simulink model "advisordemo2"  (Simulink 5.0)
settings: Solver=FixedStepDiscrete  SolverMode=SingleTasking  StartTime=0.0  StopTime=4  FixedStep=1  RelTol=1e-3  AbsTol=1e-6
libraries: fixpt_lib_4 x4
settings Model: ExecutionOrder=on  CovMetricSettings=d  Creator=andyb  LastModifiedBy=batserve  ExtModeMexFile=no_ext_comm  ExtModeTrigMode=oneshot  ExtModeArmWhenConnect=off  ExtModeAutoUpdateStatusClock=off  RTWExpressionDepthLimit=1  SaveTime=off  SaveOutput=off  LimitDataPoints=off  IntegerOverflowMsg=none  ParameterDowncastMsg=warning  ParameterOverflowMsg=warning  ParameterPrecisionLossMsg=none  RTWInlineParameters=on  ProdHWWordLengths=8,16,16,32  RTWSystemTargetFile=ert.tlc  RTWTemplateMakefile=ert_default_tmf  RTWGenerateCodeOnly=on  RTWOptions="-aCombineOutputUpdateFcns=1 -aEnforceIntegerDowncast=0 -aExtMode=0 -aExtModeTesting=0 -aFoldNonRolledExpr=1 -aForceParamTrailComments=0 -aGenFloatMathFcnCalls=\"ANSI_C\" -aGenerateASAP2=0 -aGenerateComments=1 -aGenerateErtSFunction=0 -aGenerateReport=1 -aGenerateSampleERTMain=0 -aIgnoreCustomStorageClasses=0 -aIncDataTypeInIds=1 -aIncHierarchyInIds=1 -aIncludeMdlTerminateFcn=0 -aInitFltsAndDblsToZero=0 -aInlineInvariantSignals=1 -aInlinedPrmAccess=\"Literals\" -aInsertBlockDesc=0 -aLocalBlockOutputs=1 -aMatFileLogging=0 -aMaxRTWIdLen=31 -aMultiInstanceERTCode=0 -aPrefixModelToSubsysFcnNames=1 -aPurelyIntegerCode=0 -aRTWVerbose=1 -aRollThreshold=5 -aShowEliminatedStatements=0 -aSuppressErrorStatus=1 -aZeroExternalMemoryAtStartup=0 -aZeroInternalMemoryAtStartup=0"

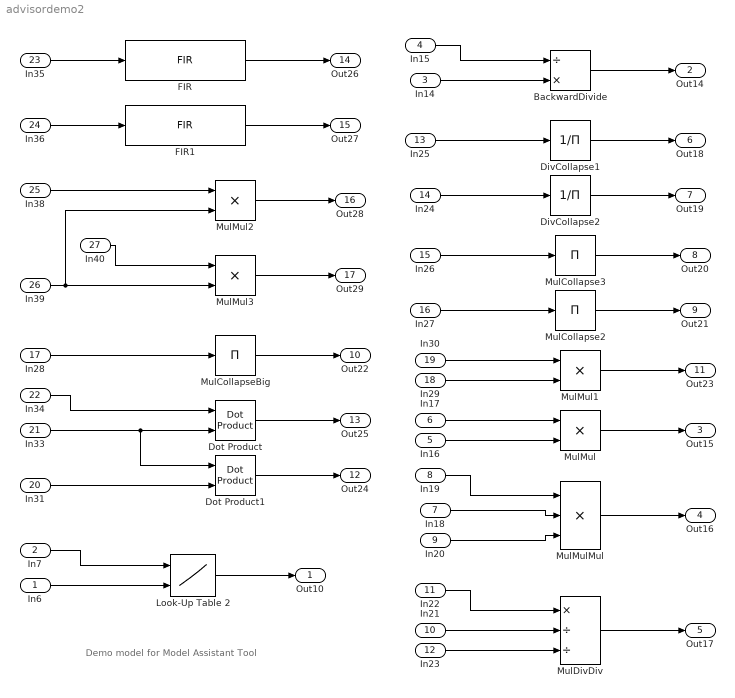
== system advisordemo2 ==
  note: Demo model for Model Assistant Tool
  In6 : Inport  PortDimensions=1  SampleTime=1  ShowAdditionalParam=on  DataType=Specify via dialog  OutScaling=2^-10  Interpolate=off
  In7 : Inport  Port=2  PortDimensions=1  SampleTime=1  ShowAdditionalParam=on  DataType=Specify via dialog  OutScaling=2^-10  Interpolate=off
  In14 : Inport  Port=3  PortDimensions=1  SampleTime=1  ShowAdditionalParam=on  DataType=Specify via dialog  OutScaling=2^-10  Interpolate=off
  In15 : Inport  Port=4  PortDimensions=1  SampleTime=1  ShowAdditionalParam=on  DataType=Specify via dialog  OutScaling=2^-10  Interpolate=off
  In16 : Inport  Port=5  PortDimensions=1  SampleTime=1  ShowAdditionalParam=on  DataType=Specify via dialog  OutDataType=sfix(32)  OutScaling=2^-10  Interpolate=off
  In17 : Inport  Port=6  PortDimensions=1  SampleTime=1  ShowAdditionalParam=on  DataType=Specify via dialog  OutScaling=2^-10  Interpolate=off
  In18 : Inport  Port=7  PortDimensions=1  SampleTime=1  ShowAdditionalParam=on  DataType=Specify via dialog  OutScaling=2^-10  Interpolate=off
  In19 : Inport  Port=8  PortDimensions=1  SampleTime=1  ShowAdditionalParam=on  DataType=Specify via dialog  OutScaling=2^-10  Interpolate=off
  In20 : Inport  Port=9  PortDimensions=1  SampleTime=1  ShowAdditionalParam=on  DataType=Specify via dialog  OutScaling=2^-10  Interpolate=off
  In21 : Inport  Port=10  PortDimensions=1  SampleTime=1  ShowAdditionalParam=on  DataType=Specify via dialog  OutScaling=2^-10  Interpolate=off
  In22 : Inport  Port=11  PortDimensions=1  SampleTime=1  ShowAdditionalParam=on  DataType=Specify via dialog  OutScaling=2^-10  Interpolate=off
  In23 : Inport  Port=12  PortDimensions=1  SampleTime=1  ShowAdditionalParam=on  DataType=Specify via dialog  OutScaling=2^-10  Interpolate=off
  In25 : Inport  Port=13  PortDimensions=1  SampleTime=1  ShowAdditionalParam=on  DataType=Specify via dialog  OutScaling=2^-10  Interpolate=off
  In24 : Inport  Port=14  PortDimensions=2  SampleTime=1  ShowAdditionalParam=on  DataType=Specify via dialog  OutScaling=2^-10  Interpolate=off
  In26 : Inport  Port=15  PortDimensions=3  SampleTime=1  ShowAdditionalParam=on  DataType=Specify via dialog  OutScaling=2^-10  Interpolate=off
  In27 : Inport  Port=16  PortDimensions=2  SampleTime=1  ShowAdditionalParam=on  DataType=Specify via dialog  OutScaling=2^-10  Interpolate=off
  In28 : Inport  Port=17  PortDimensions=2  SampleTime=1  ShowAdditionalParam=on  DataType=Specify via dialog  OutDataType=sfix(32)  OutScaling=2^-10  Interpolate=off
  In29 : Inport  Port=18  PortDimensions=1  SampleTime=1  ShowAdditionalParam=on  DataType=Specify via dialog  OutScaling=2^-10  Interpolate=off
  In30 : Inport  Port=19  PortDimensions=1  SampleTime=1  ShowAdditionalParam=on  DataType=Specify via dialog  OutScaling=2^-10  Interpolate=off
  In31 : Inport  Port=20  PortDimensions=1  SampleTime=1  ShowAdditionalParam=on  DataType=Specify via dialog  OutDataType=sfix(32)  OutScaling=2^-10  Interpolate=off
  In33 : Inport  Port=21  PortDimensions=1  SampleTime=1  ShowAdditionalParam=on  DataType=Specify via dialog  OutScaling=2^-10  Interpolate=off
  In34 : Inport  Port=22  PortDimensions=1  SampleTime=1  ShowAdditionalParam=on  DataType=Specify via dialog  OutScaling=2^-10  Interpolate=off
  In35 : Inport  Port=23  PortDimensions=1  SampleTime=1  ShowAdditionalParam=on  DataType=Specify via dialog  OutDataType=sfix(32)  OutScaling=2^-10  Interpolate=off
  In36 : Inport  Port=24  PortDimensions=1  SampleTime=1  ShowAdditionalParam=on  DataType=Specify via dialog  OutDataType=sfix(32)  OutScaling=2^-10  Interpolate=off
  In38 : Inport  Port=25  PortDimensions=1  SampleTime=1  ShowAdditionalParam=on  DataType=Specify via dialog  OutScaling=1.01 * 2^-10  Interpolate=off
  In39 : Inport  Port=26  PortDimensions=1  SampleTime=1  ShowAdditionalParam=on  DataType=Specify via dialog  OutScaling=2^-10  Interpolate=off
  In40 : Inport  Port=27  PortDimensions=1  SampleTime=1  ShowAdditionalParam=on  DataType=Specify via dialog  OutScaling=[2^-10 1]  Interpolate=off
  BackwardDivide : Product  Inputs=/*  ShowAdditionalParam=on  OutDataTypeMode=Specify via dialog  OutScaling=2^-10
  DivCollapse1 : Product  Inputs=/  ShowAdditionalParam=on  OutDataTypeMode=Specify via dialog  OutScaling=2^-10
  DivCollapse2 : Product  Inputs=/  ShowAdditionalParam=on  OutDataTypeMode=Specify via dialog  OutScaling=2^-10
  Dot Product : fixpt_lib_4/Math/Dot Product  OutputDataTypeScalingMode=Specify via dialog  OutDataType=sfix(32)  OutScaling=2^-10  DoSatur=off
  Dot Product1 : fixpt_lib_4/Math/Dot Product  OutputDataTypeScalingMode=Specify via dialog  OutDataType=sfix(32)  OutScaling=2^-10  DoSatur=off
  FIR : fixpt_lib_4/Filters/FIR  mgainval=[0.1:0.1:1 0.9:-0.1:0.1]  vinit=0.0  samptime=-1  GainDataTypeScalingMode=Specify via dialog  GainDataType=sfix( 16 )  GainScaling=2^-14  MatRadixGroup=Best Precision: Matrix-wise  OutputDataTypeScalingMode=Specify via dialog  OutDataType=sfix(32)  OutScaling=2^-10  DoSatur=off
  FIR1 : fixpt_lib_4/Filters/FIR  mgainval=[0.1:0.1:1 0.9:-0.1:0.1]  vinit=0.0  samptime=-1  GainDataTypeScalingMode=Specify via dialog  GainDataType=sfix( 16 )  GainScaling=2^-14  MatRadixGroup=Best Precision: Matrix-wise  OutputDataTypeScalingMode=Specify via dialog  OutDataType=sfix(32)  OutScaling=2^-20  DoSatur=off
  Look-Up Table 2 : Lookup2D  RowIndex=[1:3]  ColumnIndex=[1 2 7]  OutputValues=[4 5 6;16 19 20;10 18 23]  ShowAdditionalParam=on  LookUpMeth=Interpolation-Use End Values  OutDataTypeMode=Specify via dialog  OutScaling=2^-10
  MulCollapse2 : Product  Inputs=1  ShowAdditionalParam=on  OutDataTypeMode=Specify via dialog  OutScaling=2^-10
  MulCollapse3 : Product  Inputs=*  ShowAdditionalParam=on  OutDataTypeMode=Specify via dialog  OutScaling=2^-10
  MulCollapseBig : Product  Inputs=1  ShowAdditionalParam=on  OutDataTypeMode=Specify via dialog  OutScaling=2^-10
  MulDivDiv : Product  Inputs=*//  ShowAdditionalParam=on  OutDataTypeMode=Specify via dialog  OutScaling=2^-10
  MulMul : Product  ShowAdditionalParam=on  OutDataTypeMode=Specify via dialog  OutScaling=2^-3
  MulMul1 : Product  ShowAdditionalParam=on  OutDataTypeMode=Specify via dialog  OutScaling=2^-10
  MulMul2 : Product  ShowAdditionalParam=on  OutDataTypeMode=Specify via dialog  OutScaling=2^-10
  MulMul3 : Product  ShowAdditionalParam=on  OutDataTypeMode=Specify via dialog  OutScaling=2^-10
  MulMulMul : Product  Inputs=3  ShowAdditionalParam=on  OutDataTypeMode=Specify via dialog  OutScaling=2^-10
  Out10 : Outport
  Out14 : Outport  Port=2
  Out15 : Outport  Port=3
  Out16 : Outport  Port=4
  Out17 : Outport  Port=5
  Out18 : Outport  Port=6
  Out19 : Outport  Port=7
  Out20 : Outport  Port=8
  Out21 : Outport  Port=9
  Out22 : Outport  Port=10
  Out23 : Outport  Port=11
  Out24 : Outport  Port=12
  Out25 : Outport  Port=13
  Out26 : Outport  Port=14
  Out27 : Outport  Port=15
  Out28 : Outport  Port=16
  Out29 : Outport  Port=17
  wires:
  In6/1 -> Look-Up Table 2/2
  Look-Up Table 2/1 -> Out10/1
  In7/1 -> Look-Up Table 2/1
  In14/1 -> BackwardDivide/2
  BackwardDivide/1 -> Out14/1
  In15/1 -> BackwardDivide/1
  MulMul/1 -> Out15/1
  In17/1 -> MulMul/1
  In18/1 -> MulMulMul/2
  MulMulMul/1 -> Out16/1
  In19/1 -> MulMulMul/1
  In20/1 -> MulMulMul/3
  In21/1 -> MulDivDiv/2
  MulDivDiv/1 -> Out17/1
  In22/1 -> MulDivDiv/1
  In23/1 -> MulDivDiv/3
  DivCollapse1/1 -> Out18/1
  In25/1 -> DivCollapse1/1
  DivCollapse2/1 -> Out19/1
  In24/1 -> DivCollapse2/1
  MulCollapse3/1 -> Out20/1
  In26/1 -> MulCollapse3/1
  MulCollapse2/1 -> Out21/1
  In27/1 -> MulCollapse2/1
  MulCollapseBig/1 -> Out22/1
  In28/1 -> MulCollapseBig/1
  MulMul1/1 -> Out23/1
  In30/1 -> MulMul1/1
  In31/1 -> Dot Product1/2
  Dot Product1/1 -> Out24/1
  In33/1 -> Dot Product/2, Dot Product1/1
  Dot Product/1 -> Out25/1
  In34/1 -> Dot Product/1
  In35/1 -> FIR/1
  FIR/1 -> Out26/1
  In36/1 -> FIR1/1
  FIR1/1 -> Out27/1
  MulMul2/1 -> Out28/1
  In38/1 -> MulMul2/1
  In39/1 -> MulMul3/2, MulMul2/2
  MulMul3/1 -> Out29/1
  In40/1 -> MulMul3/1
  In16/1 -> MulMul/2
  In29/1 -> MulMul1/2
